simulink model "Practica4_Observador"  (R2022a)
settings: Solver=ode4  StartTime=0.0  StopTime=15  FixedStep=0.001  RelTol=1e-3
model workspace (MAT data in the model file):
  ci = 700
settings Model: Creator=edgar  LastModifiedBy=Anahi Monserrat
settings ModelReferenceCC: EnableRefExpFcnMdlSchedulingChecks=off
settings RTWCC: Description=Generic Real-Time Target

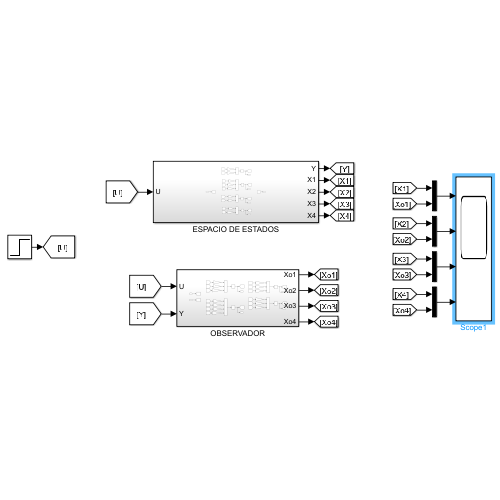
[thumbnail: Simulink's stored preview of the top-level diagram]
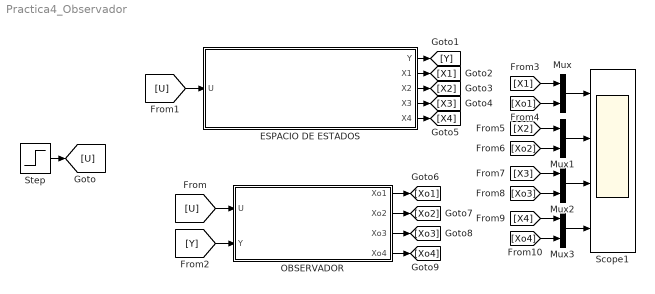
== system Practica4_Observador ==
  ESPACIO DE ESTADOS : Subsystem
  Mux{,1..3} (4 alike) : Mux  Inputs=2
  OBSERVADOR : Subsystem
  Scope1 : Scope  NumInputPorts=4
  Step : Step  SampleTime=0
  wires:
  Step/1 -> [U]
  [U] -> OBSERVADOR/1(U)
  [U] -> ESPACIO DE ESTADOS/1(U)
  ESPACIO DE ESTADOS/1(Y) -> [Y]
  ESPACIO DE ESTADOS/2(X1) -> [X1]
  ESPACIO DE ESTADOS/3(X2) -> [X2]
  ESPACIO DE ESTADOS/4(X3) -> [X3]
  ESPACIO DE ESTADOS/5(X4) -> [X4]
  OBSERVADOR/1(Xo1) -> [Xo1]
  OBSERVADOR/2(Xo2) -> [Xo2]
  OBSERVADOR/4(Xo4) -> [Xo4]
  OBSERVADOR/3(Xo3) -> [Xo3]
  Mux/1 -> Scope1/1
  Mux1/1 -> Scope1/2
  Mux2/1 -> Scope1/3
  Mux3/1 -> Scope1/4
  [Y] -> OBSERVADOR/2(Y)
  [X1] -> Mux/1
  [Xo1] -> Mux/2
  [X2] -> Mux1/1
  [Xo2] -> Mux1/2
  [X3] -> Mux2/1
  [Xo3] -> Mux2/2
  [X4] -> Mux3/1
  [Xo4] -> Mux3/2

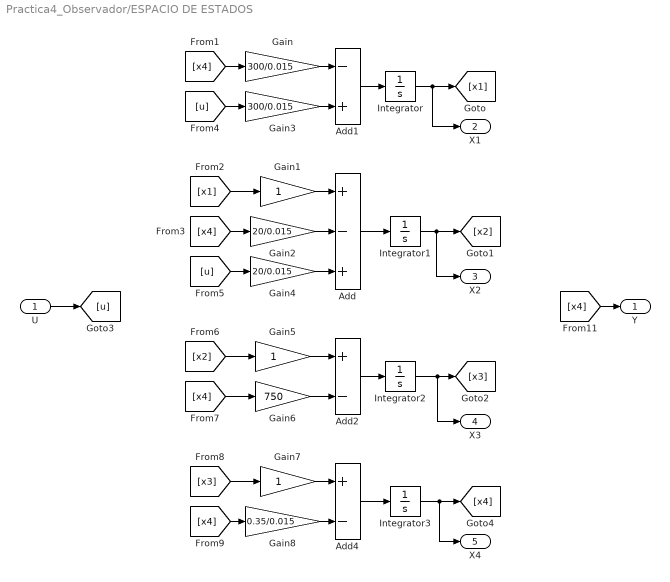
== system Practica4_Observador/ESPACIO DE ESTADOS ==
  U : Inport
  Add : Sum  Inputs=+-+
  Add1 : Sum  Inputs=-+
  Add2 : Sum  Inputs=+-
  Add4 : Sum  Inputs=+-
  Gain : Gain  Gain=300/0.015
  Gain1 : Gain
  Gain2 : Gain  Gain=20/0.015
  Gain3 : Gain  Gain=300/0.015
  Gain4 : Gain  Gain=20/0.015
  Gain5 : Gain
  Gain6 : Gain  Gain=750
  Gain7 : Gain
  Gain8 : Gain  Gain=0.35/0.015
  Integrator : Integrator  InitialCondition=ci
  Integrator1 : Integrator  InitialCondition=250
  Integrator2 : Integrator  InitialCondition=ci
  Integrator3 : Integrator  InitialCondition=ci
  Y : Outport
  X1 : Outport  Port=2
  X2 : Outport  Port=3
  X3 : Outport  Port=4
  X4 : Outport  Port=5
  wires:
  Integrator/1 -> X1/1, [x1]
  U/1 -> [u]
  [x4] -> Gain/1
  [x1] -> Gain1/1
  Integrator1/1 -> X2/1, [x2]
  Add/1 -> Integrator1/1
  Gain1/1 -> Add/1
  [x4] -> Gain2/1
  Gain2/1 -> Add/2
  Add1/1 -> Integrator/1
  Gain/1 -> Add1/1
  [u] -> Gain3/1
  Gain3/1 -> Add1/2
  [u] -> Gain4/1
  Gain4/1 -> Add/3
  Gain6/1 -> Add2/2
  [x4] -> Gain6/1
  Gain5/1 -> Add2/1
  Add2/1 -> Integrator2/1
  [x2] -> Gain5/1
  Integrator2/1 -> X3/1, [x3]
  Gain8/1 -> Add4/2
  [x4] -> Gain8/1
  Gain7/1 -> Add4/1
  Add4/1 -> Integrator3/1
  Integrator3/1 -> X4/1, [x4]
  [x3] -> Gain7/1
  [x4] -> Y/1

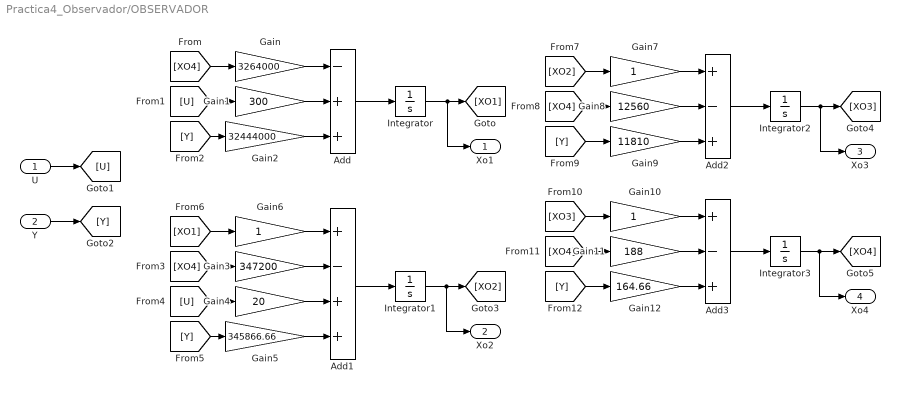
== system Practica4_Observador/OBSERVADOR ==
  U : Inport
  Y : Inport  Port=2
  Add : Sum  Inputs=-++
  Add1 : Sum  Inputs=+-++
  Add2 : Sum  Inputs=+-+
  Add3 : Sum  Inputs=+-+
  Gain : Gain  Gain=3264000
  Gain1 : Gain  Gain=300
  Gain10 : Gain
  Gain11 : Gain  Gain=188
  Gain12 : Gain  Gain=164.66
  Gain2 : Gain  Gain=32444000
  Gain3 : Gain  Gain=347200
  Gain4 : Gain  Gain=20
  Gain5 : Gain  Gain=345866.66
  Gain6 : Gain
  Gain7 : Gain
  Gain8 : Gain  Gain=12560
  Gain9 : Gain  Gain=11810
  Integrator{,1..3} (4 alike) : Integrator
  Xo1 : Outport
  Xo2 : Outport  Port=2
  Xo3 : Outport  Port=3
  Xo4 : Outport  Port=4
  wires:
  Add/1 -> Integrator/1
  Integrator/1 -> Xo1/1, [XO1]
  [XO4] -> Gain/1
  U/1 -> [U]
  Y/1 -> [Y]
  [U] -> Gain1/1
  Gain/1 -> Add/1
  Gain1/1 -> Add/2
  [Y] -> Gain2/1
  Gain2/1 -> Add/3
  [Y] -> Gain5/1
  [U] -> Gain4/1
  [XO4] -> Gain3/1
  Integrator1/1 -> Xo2/1, [XO2]
  Add1/1 -> Integrator1/1
  [XO1] -> Gain6/1
  Gain6/1 -> Add1/1
  Gain3/1 -> Add1/2
  Gain4/1 -> Add1/3
  Gain5/1 -> Add1/4
  Gain9/1 -> Add2/3
  [Y] -> Gain9/1
  Gain8/1 -> Add2/2
  Gain7/1 -> Add2/1
  [XO4] -> Gain8/1
  [XO2] -> Gain7/1
  Integrator2/1 -> Xo3/1, [XO3]
  Add2/1 -> Integrator2/1
  Add3/1 -> Integrator3/1
  Integrator3/1 -> Xo4/1, [XO4]
  [XO3] -> Gain10/1
  [XO4] -> Gain11/1
  Gain10/1 -> Add3/1
  Gain11/1 -> Add3/2
  [Y] -> Gain12/1
  Gain12/1 -> Add3/3
